simulink model "ICN_with_BR_input_model4test_clusterParams_PF2C_NLR"  (R2020b)
settings: Solver=ode15s  StartTime=0.5  StopTime=1080  RelTol=1e-3  EnableMultiTasking=on
model workspace (MAT data in the model file):
  HRResponseIano = [1 0.976355617701 1.05061592575 1.14391807051 1.22959062218 1.30026078221 1.35513299833 1.39551709306 1.423380234 1.44057518669 1.44870724956 1.44945189675 ... (1201 elements, 1x1201)]
values from neighbouring files (symbols this model uses):
  LBNP_input = Simulink.Parameter(LBNP_input)    [BRclosedLoop_model_initialize_params.m]
libraries: simulink x1
(part 3 of 3)

== system ICN_with_BR_input_model4test_clusterParams_PF2C_NLR/Autonomic Nervous System/ICN/PN-DMV/midptDMV_PN1 ==
  Divide : Product  Inputs=**
  Sum : Sum  Inputs=|++
  midptDMV_PN_gain : Constant  Value=0.7
  Out1 : Outport
  wires:
  Divide/1 -> Out1/1
  [maxout_LCN] -> Sum/1
  [maxout_fevEmax] -> Sum/2
  Sum/1 -> Divide/2
  midptDMV_PN_gain/1 -> Divide/1

== system ICN_with_BR_input_model4test_clusterParams_PF2C_NLR/Autonomic Nervous System/ICN/PN-NA/midptNA_PN1 ==
  Divide : Product  Inputs=**
  Scope : Scope
  Sum : Sum  Inputs=|++
  midptNA_PN_gain : Constant
  Out1 : Outport
  wires:
  midptNA_PN_gain/1 -> Divide/1
  Sum/1 -> Divide/2
  [maxout_fevHR] -> Scope/1, Sum/2
  [maxout_LCN] -> Sum/1
  Divide/1 -> Out1/1
